simulink model "simulation_gripen_regulation"  (R2022b)
settings: Solver=ode15s  StartTime=0.0  StopTime=200  RelTol=1e-3  EnableMultiTasking=on
values from neighbouring files (symbols this model uses):
  A = [-0.292 -0.152 0.0364 0 0 0 0 8.13 -2.54 -0.0678 1 0 ... (49 elements, 7x7)]    [Gripendata.mat]
  B = [0 -31.7 0 0 0 20 0 -2.15 0.0274 1.48 0 0 ... (14 elements, 7x2)]    [Gripendata.mat]
  C = [0 0 0 0 0 0 1 0 0 1 0 0 ... (14 elements, 2x7)]    [Gripendata.mat]
  D = [0  0; 0  0]    [Gripendata.mat]
  x0 = [5 0.00174532925199 0.00174532925199 0.0872664625997 0.0872664625997 0 0]    [Gripendata.mat]
undefined symbols (not defined in the file or in its folder): A_ob, B_ob, C_ob, D_ob, Kpp
settings Model: Creator=scattolini  LastModifiedBy=marco
settings SolverCC: AlgebraicLoopSolver=TrustRegion
settings DataIOCC: LimitDataPoints=on  SaveFormat=Array  SignalLoggingSaveFormat=ModelDataLogs  ReturnWorkspaceOutputs=off
settings OptimizationCC: ExpressionDepthLimit=2147483647  InitFltsAndDblsToZero=on  LifeSpan=inf
settings DebuggingCC: SaveWithParameterizedLinksMsg=none  UnderspecifiedInitializationDetection=Classic  MergeDetectMultiDrivingBlocksExec=none  SignalResolutionControl=TryResolveAllWithWarning  SolverPrmCheckMsg=warning  MultiTaskDSMMsg=warning  MultiTaskCondExecSysMsg=none  FcnCallInpInsideContextMsg=warning  UnconnectedInputMsg=warning  UnconnectedOutputMsg=warning  UnconnectedLineMsg=warning  StateNameClashWarn=warning  SFUnexpectedBacktrackingDiag=warning  SFNoUnconditionalDefaultTransitionDiag=warning  SFExecutionAtInitializationDiag=none  SFMachineParentedDataDiag=warning  ArithmeticOperatorsInVariantConditions=warning
settings HardwareCC: ProdBitPerPointer=32  ProdBitPerSizeT=32  ProdBitPerPtrDiffT=32  ProdLargestAtomicFloat=None  ProdIntDivRoundTo=Undefined  ProdEndianess=Unspecified  ProdWordSize=32  ProdHWDeviceType=32-bit Generic
settings ModelReferenceCC: EnableRefExpFcnMdlSchedulingChecks=on  PropagateSignalLabelsOutOfModel=off
settings SFSimCC: SimUseLocalCustomCode=off  CustomCodeUndefinedFunction=UseInterfaceOnly
settings RTWCC: RTWUseLocalCustomCode=off  DLArmComputeVersion=19.05
settings CodeAppCC: StateflowObjectComments=on
settings GRTTargetCC: TargetFcnLib=ansi_tfl_tmw.mat  TargetLangStandard=C89/C90 (ANSI)  CombineOutputUpdateFcns=off  GRTInterface=on
settings ConfigComp: CovMetricSettings=dw  CovSaveCumulativeToWorkspaceVar=on  CovSaveSingleToWorkspaceVar=on  CovExternalEMLEnable=off

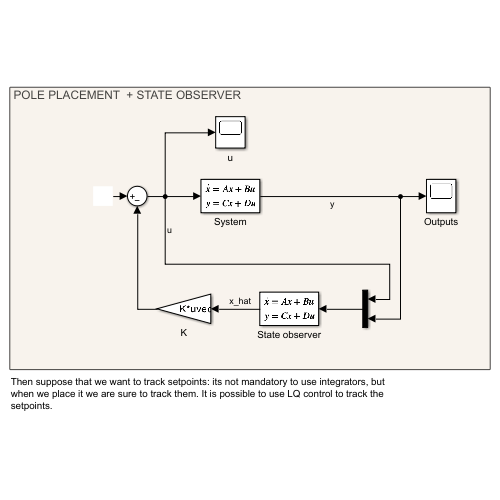
[thumbnail: Simulink's stored preview of the top-level diagram]
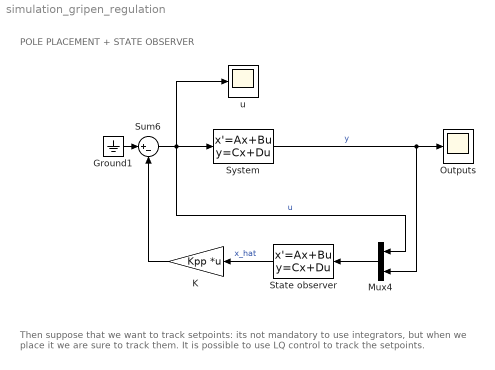
== system simulation_gripen_regulation ==
  note: Then suppose that we want to track setpoints: its not mandatory to use integrators, but when we place it we are sure to track them. It is possible to use LQ control to track the setpoints.
  note: POLE PLACEMENT + STATE OBSERVER
  Ground1 : Ground
  K : Gain  Gain=Kpp  Multiplication=Matrix(K*u) (u vector)
  Mux4 : Mux  Inputs=2
  Outputs : Scope
  State observer : StateSpace  A=A_ob  B=B_ob  C=C_ob  D=D_ob  InitialCondition=0
  Sum6 : Sum  Inputs=|+-
  System : StateSpace  A=A  B=B  C=C  D=D  InitialCondition=x0
  u : Scope
  wires:
  Ground1/1 -> Sum6/1
  Sum6/1 -> u/1, Mux4/1, System/1  "u"
  System/1 -> Mux4/2, Outputs/1  "y"
  K/1 -> Sum6/2
  Mux4/1 -> State observer/1
  State observer/1 -> K/1  "x_hat"
